simulink model "identyfikacja"  (R2022b)
settings: Solver=VariableStepAuto  StartTime=0.0  StopTime=tmax  MaxStep=5  RelTol=1e-3
values from neighbouring files (symbols this model uses):
  dFmw = 0.1*FmgN    (= 0.01)    [obliczenia.m]    (also in obliczenia2.m = 0)
  k1 = (20.2553 - 20)/dFmw    (= 25.53)    [obliczenia.m]    (also in obliczenia2.m = 65.8)
  k2 = (20.2553 - 20)/dFmw    (= 25.53)    [obliczenia.m]
  Tczas1 = 25390-Topu1    (= 21570)    [obliczenia.m]    (also in obliczenia2.m = 12463)
  Tczas2 = 21425-11955    (= 9470)    [obliczenia.m]
  Topu1 = 5820- tsok    (= 3820)    [obliczenia.m]    (also in obliczenia2.m = 1080)
  Topu2 = 21425 - Tczas2    (= 11955)    [obliczenia.m]
  tsok = 2000    [obliczenia.m]    (also in obliczenia2.m = 80000)
  TwewN = 20    [obliczenia.m]    (also in obliczenia2.m)
settings Model: Creator=asialalala  LastModifiedBy=asialalala
settings DataIOCC: ReturnWorkspaceOutputs=off

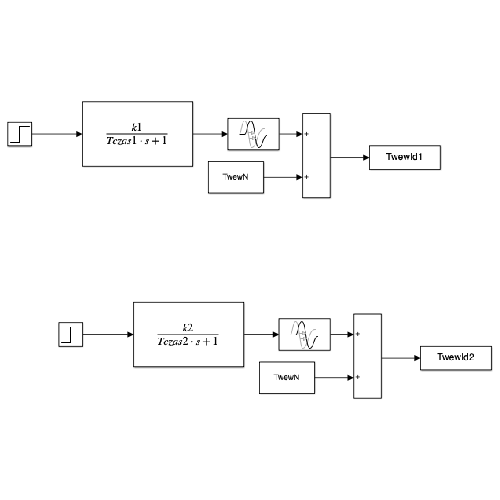
[thumbnail: Simulink's stored preview of the top-level diagram]
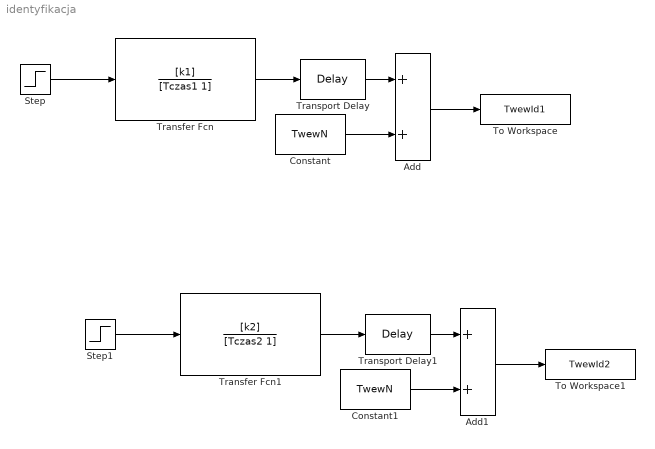
== system identyfikacja ==
  Add : Sum
  Add1 : Sum
  Constant : Constant  Value=TwewN
  Constant1 : Constant  Value=TwewN
  Step : Step  Time=tsok  After=dFmw  SampleTime=0
  Step1 : Step  Time=tsok  After=dFmw  SampleTime=0
  To Workspace : ToWorkspace  VariableName=TwewId1  SampleTime=-1
  To Workspace1 : ToWorkspace  VariableName=TwewId2  SampleTime=-1
  Transfer Fcn : TransferFcn  Numerator=[k1]  Denominator=[Tczas1 1]
  Transfer Fcn1 : TransferFcn  Numerator=[k2]  Denominator=[Tczas2 1]
  Transport Delay : TransportDelay  DelayTime=Topu1
  Transport Delay1 : TransportDelay  DelayTime=Topu2
  wires:
  Step/1 -> Transfer Fcn/1
  Transfer Fcn/1 -> Transport Delay/1
  Constant/1 -> Add/2
  Add/1 -> To Workspace/1
  Transport Delay/1 -> Add/1
  Add1/1 -> To Workspace1/1
  Constant1/1 -> Add1/2
  Step1/1 -> Transfer Fcn1/1
  Transfer Fcn1/1 -> Transport Delay1/1
  Transport Delay1/1 -> Add1/1
